simulink model "dc_motor"  (R2013b)
settings: Solver=ode3  StartTime=0.0  StopTime=0.2  FixedStep=1e-3  RelTol=1e-3
values from neighbouring files (symbols this model uses):
  ce = (Un - In*R)/wn    (= 0.301701587302)    [params.m]    (also in params_fun.m)
  cm = Mn/In    (= 0.212068965517)    [params.m]    (also in params_fun.m)
  Jm = 0.59*10^(-4)    (= 5.9e-05)    [params.m]    (also in params_fun.m)
  L = 130*10^(-3)    (= 0.13)    [params.m]    (also in params_fun.m)
  PwrAmpl = 50    [params.m]
  R = 25.8    [params.m]    (also in params_fun.m)
  Un = 110    [params.m]    (also in params_fun.m)
settings Model: Creator=user  LastModifiedBy=user
settings DataIOCC: LimitDataPoints=off

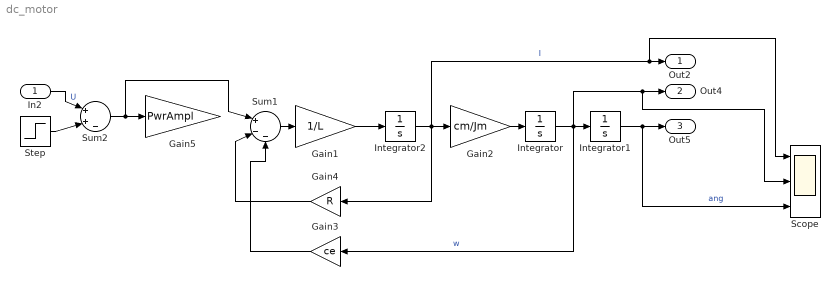
== system dc_motor ==
  In2 : Inport
  Gain1 : Gain  Gain=1/L
  Gain2 : Gain  Gain=cm/Jm
  Gain3 : Gain  Gain=ce
  Gain4 : Gain  Gain=R
  Gain5 : Gain  Gain=PwrAmpl
  Integrator : Integrator
  Integrator1 : Integrator
  Integrator2 : Integrator
  Scope : Scope  NumInputPorts=3
      settings: YMin=-5~-5~-5  YMax=5~5~5
  Step : Step  Time=0  After=Un  SampleTime=0
  Sum1 : Sum  Inputs=|+--
  Sum2 : Sum  Inputs=|++-
  Out2 : Outport
  Out4 : Outport  Port=2
  Out5 : Outport  Port=3
  wires:
  Integrator2/1 -> Gain4/1, Gain2/1, Scope/1, Out2/1  "I"
  Gain2/1 -> Integrator/1
  Integrator/1 -> Gain3/1, Scope/2, Out4/1, Integrator1/1  "w"
  Sum1/1 -> Gain1/1
  Integrator1/1 -> Scope/3, Out5/1  "ang"
  Gain1/1 -> Integrator2/1
  Gain4/1 -> Sum1/2
  Gain3/1 -> Sum1/3
  In2/1 -> Sum2/1  "U"
  Sum2/1 -> Sum1/1, Gain5/1
  Step/1 -> Sum2/2
